simulink model "PitchController"  (R2021a)
settings: Solver=ode45  StartTime=0.0  StopTime=50  RelTol=1e-3
undefined symbols (not defined in the file): servo, ThetaController_KD, ThetaController_KI, ThetaController_KP, X0
libraries: cstblocks x5, simulink_extras x4
settings Model: Creator=User01  LastModifiedBy=User01

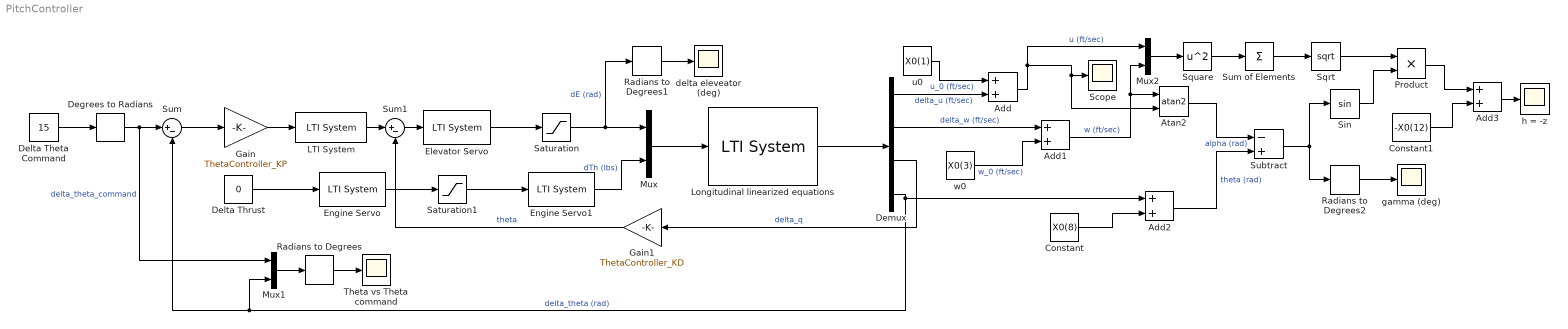
== system PitchController ==
  Add{,1..3} (4 alike) : Sum
  Atan2 : Trigonometry  Operator=atan2
  Constant : Constant  Value=X0(8)
  Constant1 : Constant  Value=-X0(12)
  Degrees to Radians : simulink_extras/Transformations/Degrees to Radians
  Delta Theta Command : Constant  Value=15
  Delta Thrust : Constant  Value=0
  Demux : Demux
  Elevator Servo : cstblocks/LTI System  sys=-servo  IC=[]
  Engine Servo : cstblocks/LTI System  sys=servo  IC=[]
  Engine Servo1 : cstblocks/LTI System  sys=servo  IC=[]
  Gain : Gain  Gain=ThetaController_KP
  Gain1 : Gain  Gain=ThetaController_KD
  LTI System : cstblocks/LTI System  sys=tf([1 ThetaController_KI/ThetaController_KP],[1 0])  IC=[]
  Longitudinal linearized equations : cstblocks/LTI System  sys=TF_long  IC=[]
  Mux : Mux  Inputs=2
  Mux1 : Mux  Inputs=2
  Mux2 : Mux  Inputs=2
  Product : Product
  Radians to Degrees : simulink_extras/Transformations/Radians to Degrees
  Radians to Degrees1 : simulink_extras/Transformations/Radians to Degrees
  Radians to Degrees2 : simulink_extras/Transformations/Radians to Degrees
  Saturation : Saturate  UpperLimit=25*pi/180  LowerLimit=-25*pi/180
  Saturation1 : Saturate  UpperLimit=25*pi/180  LowerLimit=-25*pi/180
  Scope : Scope
  Sin : Trigonometry
  Sqrt : Sqrt  SaturateOnIntegerOverflow=on
  Square : Math  Operator=square  SaturateOnIntegerOverflow=on
  Subtract : Sum  Inputs=-+
  Sum : Sum  Inputs=|+-
  Sum of Elements : Sum  Inputs=+
  Sum1 : Sum  Inputs=|+-
  Theta vs Theta command : Scope
  delta eleveator (deg) : Scope
  gamma (deg) : Scope
  h = -z : Scope
  u0 : Constant  Value=X0(1)
  w0 : Constant  Value=X0(3)
  wires:
  Gain/1 -> LTI System/1
  Demux/3 -> Gain1/1  "delta_q"
  Delta Theta Command/1 -> Degrees to Radians/1
  Sum/1 -> Gain/1
  Degrees to Radians/1 -> Mux1/1, Sum/1  "delta_theta_command"
  Gain1/1 -> Sum1/2  "theta"
  Longitudinal linearized equations/1 -> Demux/1
  Delta Thrust/1 -> Engine Servo/1
  Engine Servo1/1 -> Mux/2  "dTh (lbs)"
  Engine Servo/1 -> Saturation1/1
  Saturation1/1 -> Engine Servo1/1
  Saturation/1 -> Radians to Degrees1/1, Mux/1  "dE (rad)"
  Elevator Servo/1 -> Saturation/1
  Mux/1 -> Longitudinal linearized equations/1
  Mux1/1 -> Radians to Degrees/1
  Radians to Degrees/1 -> Theta vs Theta command/1
  Demux/4 -> Add2/1, Sum/2, Mux1/2  "delta_theta (rad)"
  Sum1/1 -> Elevator Servo/1
  LTI System/1 -> Sum1/1
  Radians to Degrees1/1 -> delta eleveator (deg)/1
  u0/1 -> Add/1  "u_0 (ft/sec)"
  Demux/1 -> Add/2  "delta_u (ft/sec)"
  Add/1 -> Atan2/2, Scope/1, Mux2/1  "u (ft/sec)"
  Add1/1 -> Atan2/1, Mux2/2  "w (ft/sec)"
  Demux/2 -> Add1/1  "delta_w (ft/sec)"
  w0/1 -> Add1/2  "w_0 (ft/sec)"
  Constant/1 -> Add2/2
  Atan2/1 -> Subtract/1  "alpha (rad)"
  Add2/1 -> Subtract/2  "theta (rad)"
  Radians to Degrees2/1 -> gamma (deg)/1
  Subtract/1 -> Radians to Degrees2/1, Sin/1
  Mux2/1 -> Square/1
  Square/1 -> Sum of Elements/1
  Sum of Elements/1 -> Sqrt/1
  Sqrt/1 -> Product/1
  Sin/1 -> Product/2
  Add3/1 -> h = -z/1
  Product/1 -> Add3/1
  Constant1/1 -> Add3/2
